simulink model "ESE4481_hw4_simulink_restored_from_autosave"  (R2021a)
settings: Solver=VariableStepAuto  StartTime=0.0  StopTime=10  RelTol=1e-3
values from neighbouring files (symbols this model uses):
  K_A = place(A_aileron, B_aileron, [-2,-4,-1])    [ESE4481_hw4_poleplacement.m]
  K_E = place(A_elevator, B_elevator, [-2,-4,-1])    [ESE4481_hw4_poleplacement.m]
  K_R = place(A_rudder, B_rudder, [-2,-4])    [ESE4481_hw4_poleplacement.m]
  K_T = place(A_throttle, B_throttle, [-2,-4])    [ESE4481_hw4_poleplacement.m]
undefined symbols (not defined in the file or in its folder): cmd_0, cmd_step, coeffs, F_aileron, F_elevator, F_hover, F_rudder, F_throttle, g, J, J_inv, J_p, m, M_inv, omega_0, p_ned_0, Theta_0, theta_hover, V_b_0
libraries: vrlib x2
settings Model: Creator=tomwh  LastModifiedBy=Liza
settings DataIOCC: ExternalInput=F_b,omega_bE,M_b

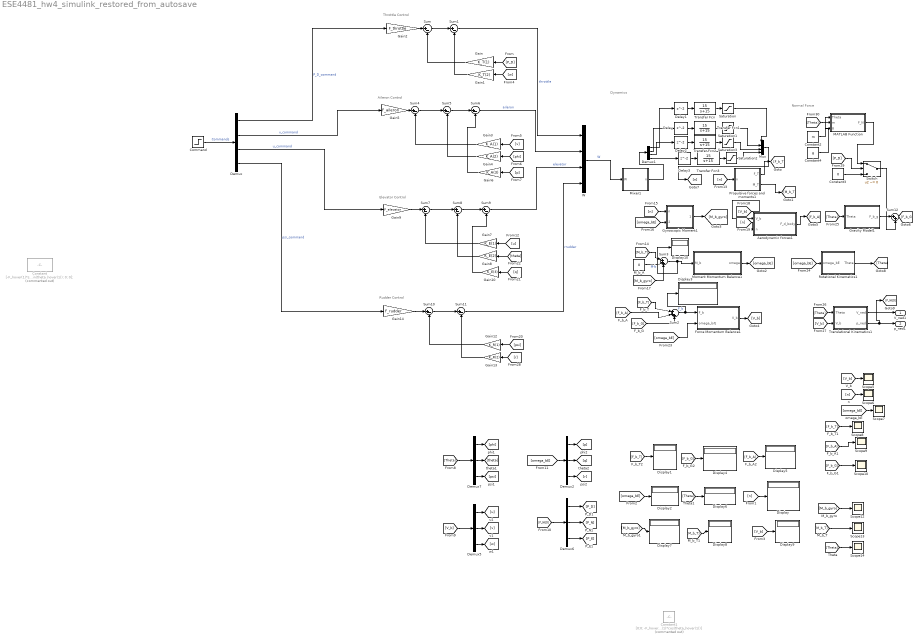
== system ESE4481_hw4_simulink_restored_from_autosave ==
  note: Normal Force
  note: Rudder Control
  note: Elevator Control
  note: Aileron Control
  note: Throttle Control
  note: Dynamics
  Aerodynamic forces1 : Subsystem
  Command : Step  Time=5  Before=cmd_0  After=cmd_step  SampleTime=0
  Constant : Constant  Commented=on  Value=[-F_hover(1)*sin(theta_hover(1)); 0; 0];
  Constant1 : Constant  Commented=on  Value=[0;0; -F_hover(1)*cos(theta_hover(1))]
  Constant2 : Constant  Value=m
  Constant3 : Constant  Value=0
  Constant4 : Constant  Value=g
  Delay{,1..3} (4 alike) : Delay  SampleTime=1/200
  Demux : Demux
  Demux1 : Demux
  Demux{2,5..7} (4 alike) : Demux  Outputs=3
  Display{,1..10} (11 alike) : Display
  Force Momentum Balance1 : Subsystem
  Gain : Gain  Gain=K_T(1)
  Gain1 : Gain  Gain=K_T(2)
  Gain10 : Gain  Gain=K_E(3)
  Gain12 : Gain  Gain=K_R(1)
  Gain13 : Gain  Gain=K_R(2)
  Gain14 : Gain  Gain=F_rudder
  Gain2 : Gain  Gain=F_throttle
  Gain3 : Gain  Gain=K_A(1)
  Gain4 : Gain  Gain=K_A(2)
  Gain5 : Gain  Gain=F_aileron
  Gain6 : Gain  Gain=K_A(3)
  Gain7 : Gain  Gain=K_E(1)
  Gain8 : Gain  Gain=K_E(2)
  Gain9 : Gain  Gain=F_elevator
  Gravity Model1 : Subsystem
  Gyroscopic Moment1 : Subsystem
  MATLAB Function : MATLAB Function  TreatAsAtomicUnit=on
  M_b_A : Constant  Value=0
  Mixer1 : Subsystem
  Moment Momentum Balance1 : Subsystem
  Mux : Mux
  Propulsive forces and moments1 : Subsystem
  Rotational Kinematics1 : Subsystem
  Saturation{,1..3} (4 alike) : Saturate  UpperLimit=500  LowerLimit=0
  Scope{5..10,12..14} (9 alike) : Scope
  Sum{,1,4..11} (10 alike) : Sum  Inputs=|+-
  Sum12 : Sum  Inputs=|++
  Sum2 : Sum  Inputs=|+++
  Sum3 : Sum  Inputs=|+++
  Switch : Switch  Criteria=u2 ~= 0
  Transfer Fcn{,1..3} (4 alike) : TransferFcn  Numerator=[15]  Denominator=[1 15]
  Translational Kinematics1 : Subsystem
  W : Mux
  V_ned1 : Outport
  p_ned1 : Outport  Port=2
  wires:
  [V_b] -> Scope5/1
  [n] -> Scope6/1
  [omega_bE] -> Scope7/1
  [F_b_T] -> Scope8/1
  [Theta] -> Scope14/1
  [M_b_T] -> Scope13/1
  [M_b_gyro] -> Scope12/1
  [F_b_G] -> Scope10/1
  [F_b_A] -> Scope9/1
  [n] -> Display/1
  [F_b_T] -> Display1/1
  [omega_bE] -> Display2/1
  [F_b_G] -> Display4/1
  [F_b_A] -> Display5/1
  [Theta] -> Display6/1
  [M_b_gyro] -> Display7/1
  [M_b_T] -> Display8/1
  [V_b] -> Display9/1
  Translational Kinematics1/1(V_ned) -> V_ned1/1
  Translational Kinematics1/2(p_ned) -> [P_NED], p_ned1/1
  Demux1/1 -> Delay1/1
  Saturation3/1 -> Mux/3
  Transfer Fcn2/1 -> Saturation3/1
  Saturation1/1 -> Mux/2
  Saturation2/1 -> Mux/4
  Saturation/1 -> Mux/1
  Transfer Fcn3/1 -> Saturation2/1
  Demux1/4 -> Delay3/1
  Delay3/1 -> Transfer Fcn3/1
  Demux1/3 -> Delay2/1
  Delay2/1 -> Transfer Fcn2/1
  Transfer Fcn1/1 -> Saturation1/1
  Demux1/2 -> Delay/1
  Delay/1 -> Transfer Fcn1/1
  Transfer Fcn/1 -> Saturation/1
  Delay1/1 -> Transfer Fcn/1
  [Theta] -> Gravity Model1/1(Theta)
  M_b_A/1 -> Sum3/2
  Mixer1/1(n) -> Demux1/1
  Propulsive forces and moments1/1(F_T) -> [F_b_T]
  Mux/1 -> [n]
  Rotational Kinematics1/1(Theta) -> [Theta]
  [Theta] -> Translational Kinematics1/1(Theta)
  Propulsive forces and moments1/2(M_T) -> [M_b_T]
  Gyroscopic Moment1/1(M_gyro) -> [M_b_gyro]
  [n] -> Propulsive forces and moments1/1(n)
  [F_b_G] -> Sum2/3
  [n] -> Gyroscopic Moment1/1(n)
  Force Momentum Balance1/1(V_b) -> [V_b]
  Aerodynamic forces1/1(F_d_body) -> [F_b_A]
  [omega_bE] -> Gyroscopic Moment1/2(omega_bE)
  [M_b_gyro] -> Sum3/3
  Sum3/1 -> Display10/1, Moment Momentum Balance1/1(M_b)  "M-b"
  [n] -> Aerodynamic forces1/2(n)
  [M_b_T] -> Sum3/1
  [F_b_A] -> Sum2/2
  Sum2/1 -> Display3/1, Force Momentum Balance1/1(F_b)  "F_b"
  [omega_bE] -> Force Momentum Balance1/2(omega_b/E)
  [F_b_T] -> Sum2/1
  [V_b] -> Aerodynamic forces1/1(V_b)
  W/1 -> Mixer1/1(W)  "W"
  [omega_bE] -> Rotational Kinematics1/1(omega_bE)
  Moment Momentum Balance1/1(omega) -> [omega_bE]
  [V_b] -> Translational Kinematics1/2(V_b)
  Sum1/1 -> W/1  "throttle"
  Sum/1 -> Sum1/1
  Gain1/1 -> Sum1/2
  [P_D] -> Gain/1
  Gain/1 -> Sum/2
  Gain2/1 -> Sum/1
  [w] -> Gain1/1
  Command/1 -> Demux/1  "Commands"
  Demux/1 -> Gain2/1  "P_D_command"
  Demux7/3 -> [psi]
  Demux7/2 -> [theta]
  Demux6/3 -> [P_E]
  Demux5/3 -> [w]
  Demux6/2 -> [P_N]
  Demux5/1 -> [u]
  Demux5/2 -> [v]
  Demux6/1 -> [P_D]
  Demux7/1 -> [phi]
  [Theta] -> Demux7/1
  [V_b] -> Demux5/1
  [P_NED] -> Demux6/1
  Demux2/3 -> [r]
  [omega_bE] -> Demux2/1
  Demux2/1 -> [p]
  Demux2/2 -> [q]
  Demux/2 -> Gain5/1  "v_command"
  Sum6/1 -> W/2  "aileron"
  Sum5/1 -> Sum6/1
  Sum4/1 -> Sum5/1
  Gain6/1 -> Sum6/2
  [phi] -> Gain4/1
  Gain5/1 -> Sum4/1
  Gain4/1 -> Sum5/2
  [p] -> Gain6/1
  [v] -> Gain3/1
  Gain3/1 -> Sum4/2
  Demux/3 -> Gain9/1  "u_command"
  [u] -> Gain7/1
  Gain8/1 -> Sum8/2
  [q] -> Gain10/1
  Gain10/1 -> Sum9/2
  Gain9/1 -> Sum7/1
  Gain7/1 -> Sum7/2
  Sum7/1 -> Sum8/1
  Sum9/1 -> W/3  "elevator"
  [theta] -> Gain8/1
  Sum8/1 -> Sum9/1
  Demux/4 -> Gain14/1  "psi_command"
  [psi] -> Gain12/1
  Sum11/1 -> W/4  "rrudder"
  Gain12/1 -> Sum10/2
  Gain14/1 -> Sum10/1
  Sum10/1 -> Sum11/1
  Gain13/1 -> Sum11/2
  [r] -> Gain13/1
  [P_D] -> Switch/2
  Gravity Model1/1(F_b_g) -> Sum12/1
  Constant3/1 -> Switch/3
  [Theta] -> MATLAB Function/1(Theta)
  Constant2/1 -> MATLAB Function/2(m)
  Constant4/1 -> MATLAB Function/3(g)
  MATLAB Function/1(F_N) -> Switch/1
  Switch/1 -> Sum12/2

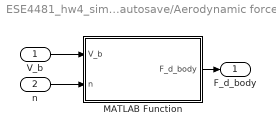
== system ESE4481_hw4_simulink_restored_from_autosave/Aerodynamic forces1 ==
  V_b : Inport
  n : Inport  Port=2
  MATLAB Function : MATLAB Function  TreatAsAtomicUnit=on
  F_d_body : Outport
  wires:
  MATLAB Function/1(F_d_body) -> F_d_body/1
  n/1 -> MATLAB Function/2(n)
  V_b/1 -> MATLAB Function/1(V_b)

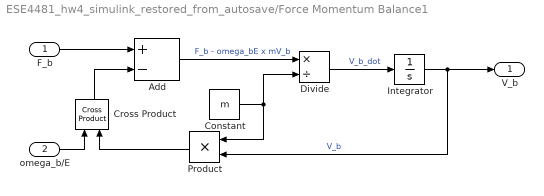
== system ESE4481_hw4_simulink_restored_from_autosave/Force Momentum Balance1 ==
  F_b : Inport
  omega_b/E : Inport  Port=2
  Add : Sum  Inputs=+-
  Constant : Constant  Value=m
  Cross Product : vrlib/Utilities/Cross Product
  Divide : Product  Inputs=*/
  Integrator : Integrator  InitialCondition=V_b_0
      settings: AttributesFormatString=%<InitialCondition>
  Product : Product
  V_b : Outport
  wires:
  omega_b/E/1 -> Cross Product/1
  F_b/1 -> Add/1
  Integrator/1 -> V_b/1, Product/2  "V_b"
  Constant/1 -> Divide/2, Product/1
  Divide/1 -> Integrator/1  "V_b_dot"
  Add/1 -> Divide/1  "F_b - omega_bE x mV_b"
  Cross Product/1 -> Add/2
  Product/1 -> Cross Product/2

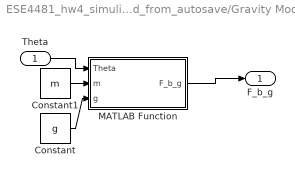
== system ESE4481_hw4_simulink_restored_from_autosave/Gravity Model1 ==
  Theta : Inport
  Constant : Constant  Value=g
  Constant1 : Constant  Value=m
  MATLAB Function : MATLAB Function  TreatAsAtomicUnit=on
  F_b_g : Outport
  wires:
  Theta/1 -> MATLAB Function/1(Theta)
  MATLAB Function/1(F_b_g) -> F_b_g/1
  Constant/1 -> MATLAB Function/3(g)
  Constant1/1 -> MATLAB Function/2(m)

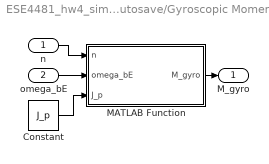
== system ESE4481_hw4_simulink_restored_from_autosave/Gyroscopic Moment1 ==
  n : Inport
  omega_bE : Inport  Port=2
  Constant : Constant  Value=J_p
  MATLAB Function : MATLAB Function  TreatAsAtomicUnit=on
  M_gyro : Outport
  wires:
  n/1 -> MATLAB Function/1(n)
  MATLAB Function/1(M_gyro) -> M_gyro/1
  omega_bE/1 -> MATLAB Function/2(omega_bE)
  Constant/1 -> MATLAB Function/3(J_p)

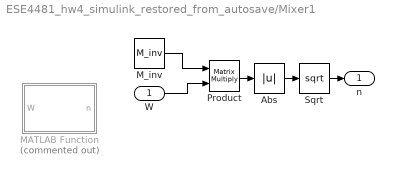
== system ESE4481_hw4_simulink_restored_from_autosave/Mixer1 ==
  W : Inport
  Abs : Abs
  MATLAB Function : MATLAB Function  Commented=on  TreatAsAtomicUnit=on
  M_inv : Constant  Value=M_inv
  Product : Product  Multiplication=Matrix(*)
  Sqrt : Sqrt  SaturateOnIntegerOverflow=on
  n : Outport
  wires:
  M_inv/1 -> Product/1
  W/1 -> Product/2
  Product/1 -> Abs/1
  Abs/1 -> Sqrt/1
  Sqrt/1 -> n/1

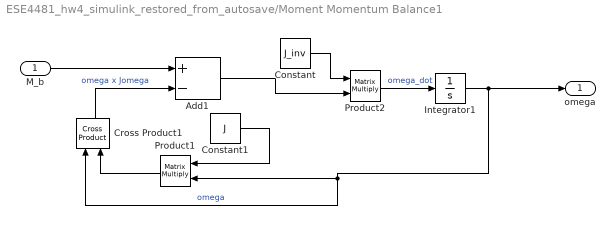
== system ESE4481_hw4_simulink_restored_from_autosave/Moment Momentum Balance1 ==
  M_b : Inport
  Add1 : Sum  Inputs=+-
  Constant : Constant  Value=J_inv
  Constant1 : Constant  Value=J
  Cross Product1 : vrlib/Utilities/Cross Product
  Integrator1 : Integrator  InitialCondition=omega_0
      settings: AttributesFormatString=%<InitialCondition>
  Product1 : Product  Multiplication=Matrix(*)
  Product2 : Product  Multiplication=Matrix(*)
  omega : Outport
  wires:
  Constant1/1 -> Product1/1
  Cross Product1/1 -> Add1/2  "omega x Jomega"
  Integrator1/1 -> omega/1, Cross Product1/1, Product1/2  "omega"
  Product1/1 -> Cross Product1/2
  Product2/1 -> Integrator1/1  "omega_dot"
  M_b/1 -> Add1/1
  Constant/1 -> Product2/1
  Add1/1 -> Product2/2

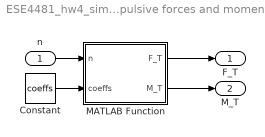
== system ESE4481_hw4_simulink_restored_from_autosave/Propulsive forces and moments1 ==
  n : Inport
  Constant : Constant  Value=coeffs
  MATLAB Function : MATLAB Function  TreatAsAtomicUnit=on
  F_T : Outport
  M_T : Outport  Port=2
  wires:
  MATLAB Function/2(M_T) -> M_T/1
  n/1 -> MATLAB Function/1(n)
  MATLAB Function/1(F_T) -> F_T/1
  Constant/1 -> MATLAB Function/2(coeffs)

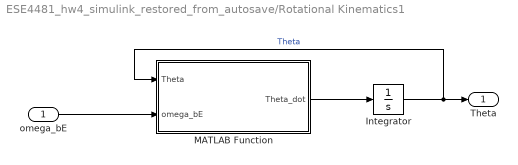
== system ESE4481_hw4_simulink_restored_from_autosave/Rotational Kinematics1 ==
  omega_bE : Inport
  Integrator : Integrator  InitialCondition=Theta_0
      settings: AttributesFormatString=%<InitialCondition>
  MATLAB Function : MATLAB Function  TreatAsAtomicUnit=on
  Theta : Outport
  wires:
  Integrator/1 -> MATLAB Function/1(Theta), Theta/1  "Theta"
  omega_bE/1 -> MATLAB Function/2(omega_bE)
  MATLAB Function/1(Theta_dot) -> Integrator/1

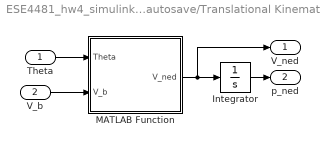
== system ESE4481_hw4_simulink_restored_from_autosave/Translational Kinematics1 ==
  Theta : Inport
  V_b : Inport  Port=2
  Integrator : Integrator  InitialCondition=p_ned_0
      settings: AttributesFormatString=%<InitialCondition>
  MATLAB Function : MATLAB Function  TreatAsAtomicUnit=on
  V_ned : Outport
  p_ned : Outport  Port=2
  wires:
  MATLAB Function/1(V_ned) -> V_ned/1, Integrator/1
  V_b/1 -> MATLAB Function/2(V_b)
  Integrator/1 -> p_ned/1
  Theta/1 -> MATLAB Function/1(Theta)

== matlab function ESE4481_hw4_simulink_restored_from_autosave/Mixer1/MATLAB Function ==
  data: W input; n output
function n = getMotorSpeeds(W)
% a = 2.034763500512882e-06;
% b = 9.690561171192599e-08;
% c = b;
% d = 1.056628184682481e-08;
rho = 1.293;
D = 0.066;
C_t = @(n) 4.375*10^(-5)*n + 0.0704; 
C_p = 0.041;
dist_xy = 0.047625; 
n_eq = 2.893014369037372e+02;
a = C_t(n_eq)*rho*D^4;
b = C_t(n_eq)*rho*D^4*dist_xy;
c = b;
d = C_p*rho*D^5/(2*pi);
M = [a a a a;
    b -b -b b;
    c c -c -c;
    -d d -d d];
nu = abs(M\W);
n = sqrt(nu);

== matlab function ESE4481_hw4_simulink_restored_from_autosave/Propulsive forces and moments1/MATLAB Function ==
  data: n input; F_T output; M_T output; coeffs input
function [F_T,M_T]= fcn(n,coeffs)
a = coeffs(1);
b = coeffs(2);
c = coeffs(3);
d = coeffs(4);
F_T = [0;0; -a*(n(1)^2 + n(2)^2 + n(3)^2 + n(4)^2)];
M_T = [b*(n(1)^2 - n(2)^2 - n(3)^2 + n(4)^2); c*(n(1)^2 + n(2)^2 - n(3)^2 - n(4)^2); d*(-n(1)^2 + n(2)^2 - n(3)^2 + n(4)^2)];

== matlab function ESE4481_hw4_simulink_restored_from_autosave/Aerodynamic forces1/MATLAB Function ==
  data: V_b input; F_d_body output; n input
function F_d_body = fcn(V_b,n)
rho = 1.293;
D = 0.066;
C_t = @(n) 4.375*10^(-5)*n + 0.0704;
K_c = 0.22;
K = [K_c 0 0;
     0 K_c 0;
     0 0 0];
F_d_body = -rho*C_t(abs(n(2)))*D^4*(n(1)^2 + n(2)^2 + n(3)^2 + n(4)^2)*K*V_b;

== matlab function ESE4481_hw4_simulink_restored_from_autosave/Gyroscopic Moment1/MATLAB Function ==
  data: n input; M_gyro output; omega_bE input; J_p input
function M_gyro = fcn(n,omega_bE,J_p)
    H = [0;0; J_p*2*pi*(n(1)-n(2)+n(3)-n(4))];
M_gyro = cross(omega_bE,H);

== matlab function ESE4481_hw4_simulink_restored_from_autosave/Gravity Model1/MATLAB Function ==
  data: Theta input; F_b_g output; m input; g input
function F_b_g = fcn(Theta,m,g)
phi = Theta(1);
theta = Theta(2);
psi = Theta(3);
R_phi = [1 0 0;
         0 cos(phi) sin(phi);
         0 -sin(phi) cos(phi)];
R_theta = [cos(theta) 0 -sin(theta);
           0 1 0;
           sin(theta) 0 cos(theta)];
R_psi = [cos(psi) sin(psi) 0;
         -sin(psi) cos(psi) 0;
         0 0 1];
R_b_E = R_phi*R_theta*R_psi;
F_b_g = R_b_E*[0; 0; m*g];

== matlab function ESE4481_hw4_simulink_restored_from_autosave/Rotational Kinematics1/MATLAB Function ==
  data: Theta input; Theta_dot output; omega_bE input
function Theta_dot = fcn(Theta,omega_bE)
    phi = Theta(1);
    theta = Theta(2);
    H_inv = [1 sin(phi)*tan(theta) cos(phi)*tan(theta);
             0 cos(phi) -sin(phi);
             0 sin(phi)*sec(theta) cos(phi)*sec(theta)];
Theta_dot = H_inv*omega_bE;

== matlab function ESE4481_hw4_simulink_restored_from_autosave/Translational Kinematics1/MATLAB Function ==
  data: Theta input; V_ned output; V_b input
function V_ned = fcn(Theta,V_b)
phi = Theta(1);
theta = Theta(2);
psi = Theta(3);
R_phi = [1 0 0;
         0 cos(phi) sin(phi);
         0 -sin(phi) cos(phi)];
R_theta = [cos(theta) 0 -sin(theta);
           0 1 0;
           sin(theta) 0 cos(theta)];
R_psi = [cos(psi) sin(psi) 0;
         -sin(psi) cos(psi) 0;
         0 0 1];
R = R_phi*R_theta*R_psi;
% R = [cos(psi)*cos(theta) cos(theta)*sin(psi) -sin(theta);
%      cos(psi)*sin(phi)*sin(theta)-cos(phi)*sin(psi) cos(phi)*cos(psi)+sin(phi)*sin(psi)*sin(theta) cos(theta)*sin(phi)
%      sin(phi)*sin(psi)+cos(phi)*cos(psi)*sin(theta) cos(phi)*sin(psi)*sin(theta)-cos(psi)*sin(phi) cos(phi)*cos(theta)];
V_ned = R\V_b;

== matlab function ESE4481_hw4_simulink_restored_from_autosave/MATLAB Function ==
  data: Theta input; F_N output; m input; g input
function F_N = fcn(Theta,m,g)
phi = Theta(1);
theta = Theta(2);
psi = Theta(3);
R_phi = [1 0 0;
         0 cos(phi) sin(phi);
         0 -sin(phi) cos(phi)];
R_theta = [cos(theta) 0 -sin(theta);
           0 1 0;
           sin(theta) 0 cos(theta)];
R_psi = [cos(psi) sin(psi) 0;
         -sin(psi) cos(psi) 0;
         0 0 1];
R_b_E = R_phi*R_theta*R_psi;
F_N = R_b_E*[0; 0; -m*g];
